simulink model "PL0_p2_ej2"  (R2022b)
settings: Solver=ode3  StartTime=0.0  StopTime=100  FixedStep=0.01  RelTol=1e-3
undefined symbols (not defined in the file or in its folder): DiscIntNeverNeededParam
libraries: simulink x2
settings Model: Creator=lucas  LastModifiedBy=lucas

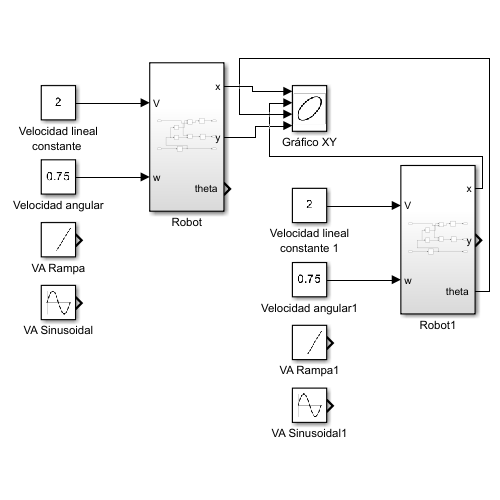
[thumbnail: Simulink's stored preview of the top-level diagram]
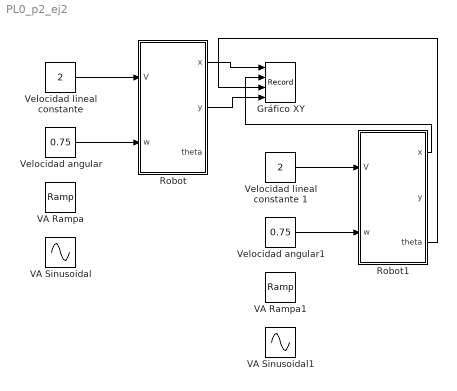
== system PL0_p2_ej2 ==
  Gráfico XY : Record  FileSettingsInternal="{\"entries\":[{\"content\":{\"excelSettings\":{\"content\":{},\"type\":\"Streamout.ExcelSettings\"}},\"type\":\"Streamout.FileSettingStorage\",\"uuid\":\"\"}],\"packageUris\":[\"http:\\/\\/schema.mathworks.com\\/mf0\\/streamout_blocks\\/R2020a\"],\"version\":\"1.0\"}"  Layout=[1 1]  SignalsInternal="{\"entries\":[{\"content\":{\"signals\":[{\"content\":{\"blockPath\":[],\"channel\":[],\"dimensions\":[1],\"domain\":\"\",\"lineColor\":\"#77ac30\",\"plots\":[1],\"port\":1,\"sid\":[\"\"],\"signalID\":2250,\"signalName\":\"Robot:1\"},\"type\":\"RecordBlkView.Signal\",\"uuid\":\"\"},{\"content\":{\"blockPath\":[],\"channel\":[],\"dimensions\":[1],\"domain\":\"\",\"lineColor\":\"#4dbeee\",\"plots\":[],\"port\":2,\"sid\":[\"\"],\"signalID\":2254,\"signalName\":\"Robot1:1\"},\"type\":\"RecordBlkView.Signal\",\"uuid\":\"\"},{\"content\":{\"blockPath\":[],\"channel\":[],\"dimensions\":[1],\"domain\":\"\",\"lineColor\":\"#edb120\",\"plots\":[],\"port\":3,\"sid\":[\"\"],\"signalID\":2258,\"signalName\":\"Robot1:3\"},\"type\":\"RecordBlkView.Signal\",\"uuid\":\"\"},{\"content\":{\"blockPath\":[],\"channel\":[],\"dimensions\":[1],\"domain\":\"\",\"lineColor\":\"#7e2f8e\",\"lineStyle\":\"DASHED\",\"plots\":[1],\"port\":4,\"sid\":[\"\"],\"signalID\":2262,\"signalName\":\"Robot:2\"},\"type\":\"RecordBlkView.Signal\",\"uuid\":\"\"}]},\"type\":\"RecordBlkView.InputSignals\",\"uuid\":\"\"}],\"packageUris\":[\"http:\\/\\/schema.mathworks.com\\/mf0\\/streamout_blocks\\/R2020a\"],\"version\":\"1.0\"}"  VisualizationBindings="{\"xyplotplugin\":{\"info\":[{\"series\":[{\"bindingParametersList\":[{\"parameter\":\"X-Axis\",\"signalID\":2250,\"signalName\":\"Robot:1\"},{\"parameter\":\"Y-Axis\",\"signalID\":2262,\"signalName\":\"Robot:2\"}],\"seriesID\":631},{\"bindingParametersList\":[{\"parameter\":\"X-Axis\",\"signalID\":2262,\"signalName\":\"Robot:2\"},{\"parameter\":\"Y-Axis\",\"signalID\":2250,\"signalName\":\"Robot:1\"}],\"seriesID\":367},{\"bindingParametersList\":[{\"parameter\":\"X-Axis\",\"signalID\":2262,\"signalName\":\"Robot:2\"}],\"seriesID\":428}],\"subplotID\":1}]}}"  CompatibilityTag=XY  st=0.01
  Robot : Subsystem
  Robot1 : Subsystem
  VA Rampa : simulink/Sources/Ramp  slope=1  start=0  InitialOutput=0
  VA Rampa1 : simulink/Sources/Ramp  slope=1  start=0  InitialOutput=0
  VA Sinusoidal : Sin  SampleTime=0
  VA Sinusoidal1 : Sin  Amplitude=2  SampleTime=0
  Velocidad angular : Constant  Value=0.75
  Velocidad angular1 : Constant  Value=0.75
  "Velocidad lineal constante " : Constant  Value=2
  Velocidad lineal constante 1 : Constant  Value=2
  wires:
  "Velocidad lineal constante "/1 -> Robot/1(V)
  Robot/1(x) -> Gráfico XY/1
  Robot/2(y) -> Gráfico XY/4
  Velocidad angular/1 -> Robot/2(w)
  Velocidad angular1/1 -> Robot1/2(w)
  Velocidad lineal constante 1/1 -> Robot1/1(V)
  Robot1/1(x) -> Gráfico XY/2
  Robot1/3("theta ") -> Gráfico XY/3

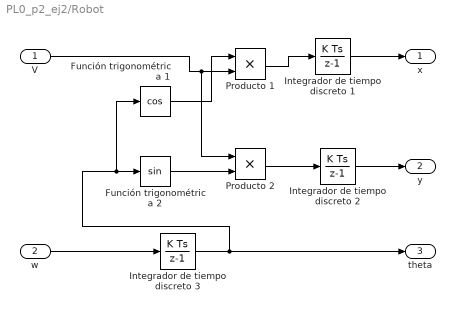
== system PL0_p2_ej2/Robot ==
  V : Inport
  w : Inport  Port=2
  Función trigonométrica 1 : Trigonometry  Operator=cos
  Función trigonométrica 2 : Trigonometry
  Integrador de tiempo discreto 1 : DiscreteIntegrator  InitialCondition=-4  SampleTime=0.01  ICPrevOutput=DiscIntNeverNeededParam  ICPrevScaledInput=DiscIntNeverNeededParam
  Integrador de tiempo discreto 2 : DiscreteIntegrator  InitialCondition=-4  SampleTime=0.01  ICPrevOutput=DiscIntNeverNeededParam  ICPrevScaledInput=DiscIntNeverNeededParam
  Integrador de tiempo discreto 3 : DiscreteIntegrator  SampleTime=0.01  ICPrevOutput=DiscIntNeverNeededParam  ICPrevScaledInput=DiscIntNeverNeededParam
  Producto 1 : Product
  Producto 2 : Product
  x : Outport  VectorParamsAs1DForOutWhenUnconnected=off
  y : Outport  Port=2  VectorParamsAs1DForOutWhenUnconnected=off
  "theta " : Outport  Port=3  VectorParamsAs1DForOutWhenUnconnected=off
  wires:
  Integrador de tiempo discreto 3/1 -> "theta "/1, Función trigonométrica 1/1, Función trigonométrica 2/1
  Función trigonométrica 1/1 -> Producto 1/1
  Producto 2/1 -> Integrador de tiempo discreto 2/1
  Producto 1/1 -> Integrador de tiempo discreto 1/1
  Integrador de tiempo discreto 1/1 -> x/1
  V/1 -> Producto 2/1, Producto 1/2
  Integrador de tiempo discreto 2/1 -> y/1
  Función trigonométrica 2/1 -> Producto 2/2
  w/1 -> Integrador de tiempo discreto 3/1

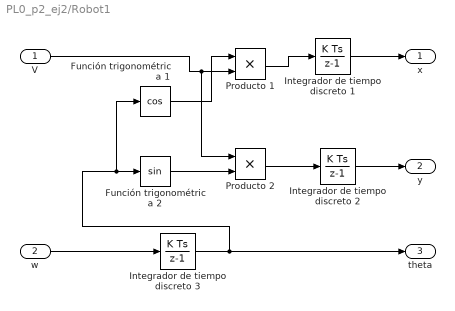
== system PL0_p2_ej2/Robot1 ==
  V : Inport
  w : Inport  Port=2
  Función trigonométrica 1 : Trigonometry  Operator=cos
  Función trigonométrica 2 : Trigonometry
  Integrador de tiempo discreto 1 : DiscreteIntegrator  SampleTime=0.01  ICPrevOutput=DiscIntNeverNeededParam  ICPrevScaledInput=DiscIntNeverNeededParam
  Integrador de tiempo discreto 2 : DiscreteIntegrator  SampleTime=0.01  ICPrevOutput=DiscIntNeverNeededParam  ICPrevScaledInput=DiscIntNeverNeededParam
  Integrador de tiempo discreto 3 : DiscreteIntegrator  SampleTime=0.01  ICPrevOutput=DiscIntNeverNeededParam  ICPrevScaledInput=DiscIntNeverNeededParam
  Producto 1 : Product
  Producto 2 : Product
  x : Outport  VectorParamsAs1DForOutWhenUnconnected=off
  y : Outport  Port=2  VectorParamsAs1DForOutWhenUnconnected=off
  "theta " : Outport  Port=3  VectorParamsAs1DForOutWhenUnconnected=off
  wires:
  Integrador de tiempo discreto 3/1 -> "theta "/1, Función trigonométrica 1/1, Función trigonométrica 2/1
  Función trigonométrica 1/1 -> Producto 1/1
  Producto 2/1 -> Integrador de tiempo discreto 2/1
  Producto 1/1 -> Integrador de tiempo discreto 1/1
  Integrador de tiempo discreto 1/1 -> x/1
  V/1 -> Producto 2/1, Producto 1/2
  Integrador de tiempo discreto 2/1 -> y/1
  Función trigonométrica 2/1 -> Producto 2/2
  w/1 -> Integrador de tiempo discreto 3/1
